simulink model "RLCircuit"  (R2020a)
settings: Solver=VariableStepAuto  StartTime=0.0  StopTime=50  RelTol=1e-3
settings Model: Creator=hp  LastModifiedBy=hp

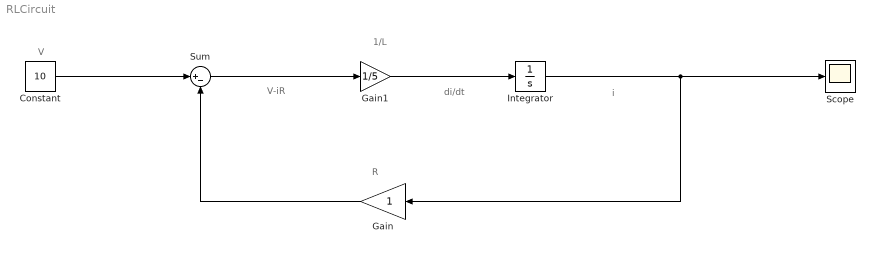
== system RLCircuit ==
  note: V
  note: V-iR
  note: 1/L
  note: R
  note: i
  note: di/dt
  Constant : Constant  Value=10
  Gain : Gain
  Gain1 : Gain  Gain=1/5
  Integrator : Integrator
  Scope : Scope
  Sum : Sum  Inputs=|+-
  wires:
  Sum/1 -> Gain1/1
  Gain1/1 -> Integrator/1
  Constant/1 -> Sum/1
  Gain/1 -> Sum/2
  Integrator/1 -> Gain/1, Scope/1
